simulink model "ModelCtrl"  (R2020b)
settings: Solver=FixedStepAuto  StartTime=0.0  StopTime=15  FixedStep=1/400  RelTol=1e-3
values from neighbouring files (symbols this model uses):
  Df = 0.011 * diag([2 1.9 0.5])    [default_parameters.m]
  fc_m = 5.0    (= 5)    [default_parameters.m]
  g = 9.81    [default_parameters.m]
  INERTIA = diag([1.0 2.0 2.5]) * 1e-4    [default_parameters.m]
  K = [-0.25 0.25 0.25 -0.25 ... (first row only)    [default_parameters.m]
  lb = [0; 0; 0; 0]    [default_parameters.m]
  MASS = 0.85    [default_parameters.m]
  MAX_ANG_ACC = 10 * diag([50.0 50.0 20.0])    [default_parameters.m]
  MAX_ESC_SPD = 6000    [default_parameters.m]
  MAX_TILT_ANGLE = 35.0    (= 35)    [default_parameters.m]
  Thrust_to_grav = 4.0    (= 4)    [default_parameters.m]
  ub = [100.0; 100.0; 100.0; 100.0]    [default_parameters.m]
  W = diag([1.0 1.0 1.0 0.5])    [default_parameters.m]
  wind_spd = [0;0;0]    [default_parameters.m]
undefined symbols (not defined in the file or in its folder): A, B, C, L
libraries: pid_lib x13, sharedtransform x6, aerolibutil x2, shared6dof x1
(part 2 of 2)

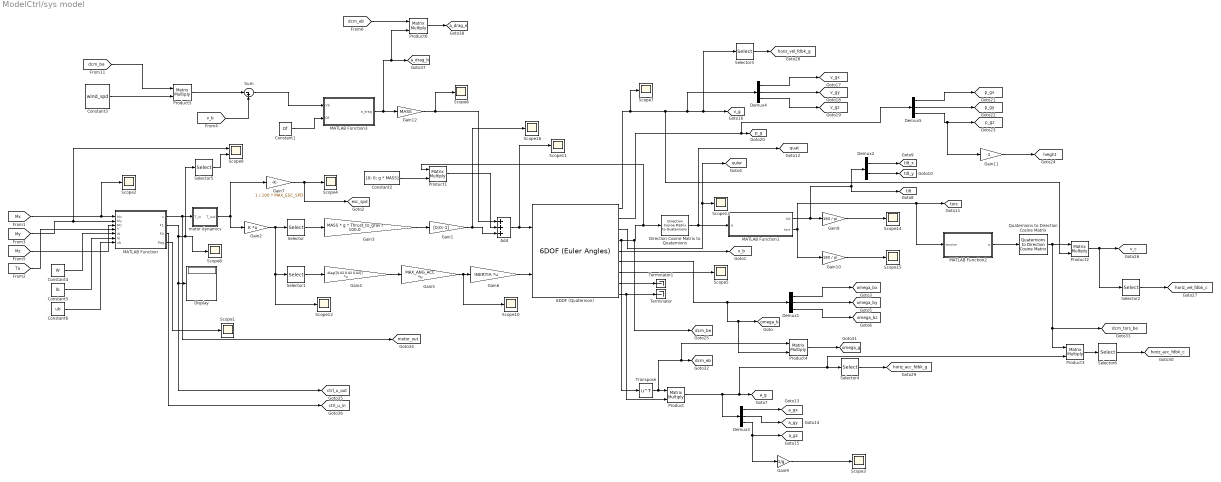
== system ModelCtrl/sys model ==
  6DOF (Quaternion) : shared6dof/6DOF (Euler Angles)  units=Metric (MKS)  mtype=Fixed  rep=Quaternion  xme_0=[0 0 0]  Vm_0=[0 0 0]  eul_0=[0 0 0]  pm_0=[0 0 0]  mass_0=MASS  mass_e=0.5  mass_f=2.0  inertia=INERTIA  inertia_e=eye(3)  inertia_f=2*eye(3)  k_quat=1.0  vre_flag=on  abi_flag=on  aMode=0  xme_statename=''  Vm_statename=''  eul_statename=''  quat_statename=''  pm_statename=''  mass_statename=''
      settings: SourceProductBaseCode=AE,PW,MT,UV,VE,VP
  Add : Sum  Inputs=+++
  Constant1 : Constant  Value=Df
  Constant2 : Constant  Value=[0; 0; g * MASS]
  Constant3 : Constant  Value=wind_spd
  Constant4 : Constant  Value=W
  Constant5 : Constant  Value=lb
  Constant6 : Constant  Value=ub
  Demux{1,3..5} (4 alike) : Demux  Outputs=3
  Demux2 : Demux  Outputs=2
  Direction Cosine Matrix to Quaternions : sharedtransform/Direction Cosine Matrix  to Quaternions  aMode=0  action=None  tolerance=eps(2)
      settings: SourceProductBaseCode=AE,PW,MT,UV,VE,VP
  Display : Display
  Gain1 : Gain  Gain=[0;0;-1]
  Gain10 : Gain  Gain=180 / pi
  Gain11 : Gain  Gain=-1
  Gain12 : Gain  Gain=MASS
  Gain2 : Gain  Gain=K  Multiplication=Matrix(K*u)
  Gain3 : Gain  Gain=MASS * g * Thrust_to_grav / 100.0
  Gain4 : Gain  Gain=diag([0.02 0.02 0.02])  Multiplication=Matrix(K*u)
  Gain5 : Gain  Gain=MAX_ANG_ACC  Multiplication=Matrix(K*u)
  Gain6 : Gain  Gain=INERTIA  Multiplication=Matrix(K*u)
  Gain7 : Gain  Gain=1 / 100 * MAX_ESC_SPD
  Gain8 : Gain  Gain=180 / pi
  Gain9 : Gain  Gain=1/g
  MATLAB Function : MATLAB Function  TreatAsAtomicUnit=on
  MATLAB Function1 : MATLAB Function  TreatAsAtomicUnit=on
  MATLAB Function2 : MATLAB Function  TreatAsAtomicUnit=on
  MATLAB Function3 : MATLAB Function  TreatAsAtomicUnit=on
  Product{,1..6} (7 alike) : Product  Multiplication=Matrix(*)
  Quaternions to Direction Cosine Matrix : sharedtransform/Quaternions to  Direction Cosine Matrix  aMode=aMode
      settings: SourceProductBaseCode=AE,PW,MT,UV,VE,VP
  Scope{1..8,10..16} (15 alike) : Scope
  Scope9 : Scope  NumInputPorts=2
  Selector : Selector  InputPortWidth=4  IndexOptions=Index vector (dialog)  Indices=[4]  OutputSizes=1
  Selector1 : Selector  InputPortWidth=4  IndexOptions=Index vector (dialog)  Indices=[1 2 3]  OutputSizes=1
  Selector{2..4,6} (4 alike) : Selector  InputPortWidth=3  IndexOptions=Index vector (dialog)  Indices=[1 2]  OutputSizes=1
  Selector5 : Selector  InputPortWidth=4  IndexOptions=Index vector (dialog)  Indices=[2]  OutputSizes=1
  Sum : Sum  Inputs=|-+
  Terminator : Terminator
  Terminator1 : Terminator
  Transpose : Math  Operator=transpose  SaturateOnIntegerOverflow=on
  motor dynamics : Subsystem
  tag scope: a_drag_b=global, a_drag_e=global, a_g=global, a_gx=global, a_gy=global, a_gz=global, ctrl_u_in=global, ctrl_u_out=global, dcm_be=global, dcm_eb=global, dcm_tors_be=global, esc_spd=global, euler=global, height=global, horiz_acc_fdbk_c=global, horiz_acc_fdbk_g=global, horiz_vel_fdbk_c=global, horiz_vel_fdbk_g=global, motor_out=global, omega_b=global, omega_bx=global, omega_by=global, omega_bz=global, omega_g=global, p_g=global, p_gx=global, p_gy=global, p_gz=global, quat=global, tilt=global, tilt_x=global, tilt_y=global, tors=global, v_b=global, v_c=global, v_g=global, v_gx=global, v_gy=global, v_gz=global
  wires:
  [Ta] -> MATLAB Function/4(T)
  [My] -> Scope9/1, MATLAB Function/2(My)
  Gain4/1 -> Gain5/1
  Gain2/1 -> Scope12/1, Selector1/1, Selector/1
  Constant5/1 -> MATLAB Function/6(lb)
  Constant6/1 -> MATLAB Function/7(ub)
  motor dynamics/1(T_out) -> Gain7/1, Gain2/1
  6DOF (Quaternion)/5 -> [v_b]
  [Mz] -> MATLAB Function/3(Mz)
  MATLAB Function1/2(tors) -> Gain10/1, MATLAB Function2/1(torsion), [tors]
  Demux1/2 -> [omega_by]
  Selector1/1 -> Gain4/1
  Selector/1 -> Gain3/1
  Demux1/3 -> [omega_bz]
  MATLAB Function/1(x) -> [motor_out], motor dynamics/1(T_in)
  Gain10/1 -> Scope15/1
  6DOF (Quaternion)/4 -> Transpose/1, [dcm_be], Product1/1, Direction Cosine Matrix to Quaternions/1
  Direction Cosine Matrix to Quaternions/1 -> [quat], MATLAB Function1/1(q)
  Gain6/1 -> 6DOF (Quaternion)/2
  [Mx] -> Scope2/1, MATLAB Function/1(Mx)
  Demux1/1 -> [omega_bx]
  6DOF (Quaternion)/3 -> [euler], Scope13/1
  Gain5/1 -> Scope10/1, Gain6/1
  Gain3/1 -> Gain1/1
  MATLAB Function/2(F1) -> [ctrl_u_out], Display/1, Selector5/1, Scope8/1
  MATLAB Function1/1(tilt) -> Demux2/1, [tilt], Gain8/1
  6DOF (Quaternion)/2 -> Demux5/1, [p_g]
  Constant4/1 -> MATLAB Function/5(W)
  Demux2/1 -> [tilt_x]
  Selector5/1 -> Scope9/2
  6DOF (Quaternion)/9 -> Product/2, Terminator/1
  6DOF (Quaternion)/8 -> Terminator1/1
  MATLAB Function/4(flag) -> Scope1/1
  Demux2/2 -> [tilt_y]
  6DOF (Quaternion)/7 -> Scope5/1
  Gain7/1 -> [esc_spd], Scope4/1
  6DOF (Quaternion)/6 -> Product4/2, [omega_b], Demux1/1
  Product/1 -> Demux3/1, Product3/2, Selector4/1, [a_g]
  Demux3/1 -> [a_gx]
  Demux3/2 -> [a_gy]
  Demux3/3 -> Gain9/1, [a_gz]
  Gain9/1 -> Scope3/1
  Gain1/1 -> Scope16/1, Add/3
  Constant2/1 -> Product1/2
  Product1/1 -> Add/2
  Demux4/1 -> [v_gx]
  Demux4/3 -> [v_gz]
  Demux4/2 -> [v_gy]
  Demux5/1 -> [p_gx]
  Demux5/2 -> [p_gy]
  Demux5/3 -> Gain11/1, [p_gz]
  Gain11/1 -> [height]
  MATLAB Function2/1(q) -> Quaternions to Direction Cosine Matrix/1
  Gain8/1 -> Scope14/1
  Quaternions to Direction Cosine Matrix/1 -> [dcm_tors_be], Product3/1, Product2/1
  6DOF (Quaternion)/1 -> Scope7/1, Selector3/1, [v_g], Demux4/1, Product2/2
  Product2/1 -> Selector2/1, [v_c]
  Selector2/1 -> [horiz_vel_fdbk_c]
  Selector3/1 -> [horiz_vel_fdbk_g]
  Selector4/1 -> [horiz_acc_fdbk_g]
  Selector6/1 -> [horiz_acc_fdbk_c]
  Product3/1 -> Selector6/1
  Add/1 -> Scope11/1, 6DOF (Quaternion)/1
  Constant1/1 -> MATLAB Function3/2(Df)
  MATLAB Function3/1(a_drag) -> Product6/2, [a_drag_b], Gain12/1
  Gain12/1 -> Scope6/1, Add/1
  Transpose/1 -> Product4/1, [dcm_eb], Product/1
  Product4/1 -> [omega_g]
  [v_b] -> Sum/2
  [dcm_be] -> Product5/1
  Constant3/1 -> Product5/2
  Product5/1 -> Sum/1
  Sum/1 -> MATLAB Function3/1(Vb)
  MATLAB Function/3(F0) -> [ctrl_u_in]
  [dcm_eb] -> Product6/1
  Product6/1 -> [a_drag_e]

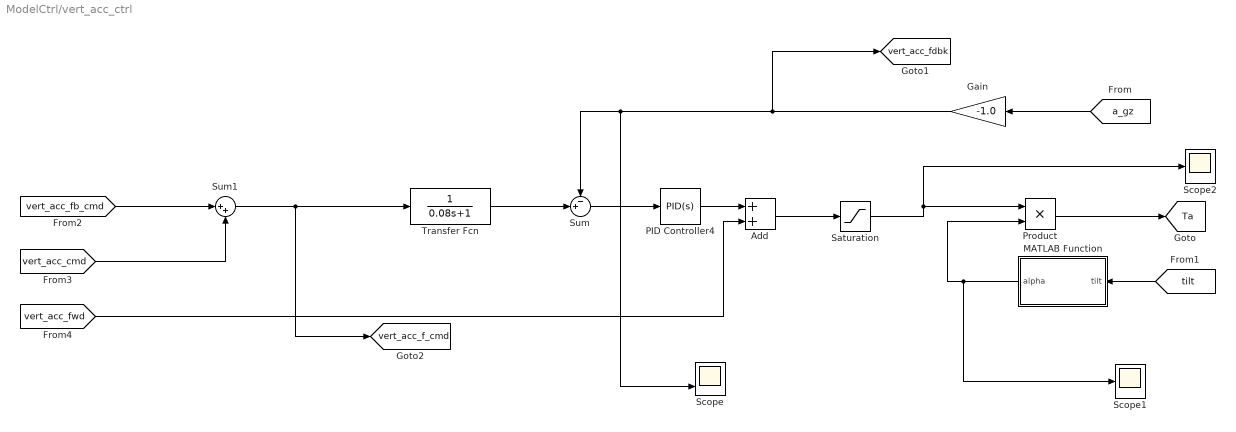
== system ModelCtrl/vert_acc_ctrl ==
  Add : Sum
  Gain : Gain  Gain=-1.0
  MATLAB Function : MATLAB Function  TreatAsAtomicUnit=on
  PID Controller4 : pid_lib/PID Controller  Controller=PID  Form=Ideal  TimeDomain=Continuous-time  UseExternalTs=off  SampleTime=-1  IntegratorMethod=Forward Euler  FilterMethod=Forward Euler  ControllerParametersSource=internal  P=35  I=10  D=0.0  UseFilter=on  N=50  TunerSelectOption=Transfer Function Based (PID Tuner App)  InitialConditionSource=internal  InitialConditionForIntegrator=0  InitialConditionForFilter=0  DifferentiatorICPrevScaledInput=0  ExternalReset=none  TrackingMode=off  Kt=1  LimitOutput=off  SatLimitsSource=internal  UpperSaturationLimit=inf  LowerSaturationLimit=-inf  LinearizeAsGain=on  AntiWindupMode=none  Kb=1  POutMin=[]  POutMax=[]  IOutMin=[]  IOutMax=[]  DOutMin=[]  DOutMax=[]  NOutMin=[]  NOutMax=[]  SumOutMin=[]  SumOutMax=[]  SaturationOutMin=[]  SaturationOutMax=[]  PParamMin=[]  PParamMax=[]  IParamMin=[]  IParamMax=[]  DParamMin=[]  DParamMax=[]  NParamMin=[]  NParamMax=[]  KbParamMin=[]  KbParamMax=[]  KtParamMin=[]  KtParamMax=[]  KbOutMin=[]  KbOutMax=[]  KtOutMin=[]  KtOutMax=[]  IntegratorOutMin=[]  IntegratorOutMax=[]  FilterOutMin=[]  FilterOutMax=[]  SumI1OutMin=[]  SumI1OutMax=[]  SumI2OutMin=[]  SumI2OutMax=[]  SumI3OutMin=[]  SumI3OutMax=[]  SumI4OutMin=[]  SumI4OutMax=[]  SumDOutMin=[]  SumDOutMax=[]  DifferentiatorOutMin=[]  DifferentiatorOutMax=[]  FilterDiffOutCoefMin=[]  FilterDiffOutCoefMax=[]  ReciprocalOutMin=[]  ReciprocalOutMax=[]  SumDenOutMin=[]  SumDenOutMax=[]  SumNumOutMin=[]  SumNumOutMax=[]  DivideOutMin=[]  DivideOutMax=[]  UdiffTsProdOutMin=[]  UdiffTsProdOutMax=[]  NTsProdOutMin=[]  NTsProdOutMax=[]  UintegralTsProdOutMin=[]  UintegralTsProdOutMax=[]  UngainTsProdOutMin=[]  UngainTsProdOutMax=[]  IntegratorContinuousStateAttributes=''  IntegratorStateMustResolveToSignalObject=off  IntegratorRTWStateStorageClass=Auto  FilterContinuousStateAttributes=''  FilterStateMustResolveToSignalObject=off  FilterRTWStateStorageClass=Auto  ParallelPVariant=Passthrough  IdealPVariant=InternalParameters  IVariant=InternalParameters  DVariant=InternalParameters  IntegratorVariant=Continuous  SatVariant=Disabled  AWVariant=Passthrough  PCopyVariant=Disabled  TRVariant=Disabled  FdbkBlocksVariant=Forward  IdealPFdbkVariant=Disabled  SatFdbkVariant=Disabled  DerivativeFilterVariant=ContFilter  NVariant=InternalParameters  NCopyVariant=Disabled  FilterICVariant=InternalICsFilter  IntegratorICVariant=InternalICs  ExternalResetVariant=Disabled  TRSumVariant=Passthrough  SumFdbkVariant=Disabled  SumVariant=Sum_PID  TsampFilterVariant=InternalTs  TsampNgainVariant=Passthrough  TsampIntegralVariant=Passthrough  ExternalSaturationOutDataTypeStr=Inherit: Same as second input
  Product : Product
  Saturation : Saturate  UpperLimit=100  LowerLimit=0
  Scope : Scope  NumInputPorts=2
  Scope1 : Scope
  Scope2 : Scope
  Sum : Sum  Inputs=-+|
  Sum1 : Sum  Inputs=|++
  Transfer Fcn : TransferFcn  Denominator=[0.08 1]
  tag scope: Ta=global, vert_acc_f_cmd=global, vert_acc_fdbk=global
  wires:
  [a_gz] -> Gain/1
  Sum/1 -> PID Controller4/1
  Gain/1 -> [vert_acc_fdbk], Sum/1, Scope/2
  [tilt] -> MATLAB Function/1(tilt)
  MATLAB Function/1(alpha) -> Scope1/1, Product/2
  Product/1 -> [Ta]
  Transfer Fcn/1 -> Sum/2
  Saturation/1 -> Scope2/1, Product/1
  PID Controller4/1 -> Add/1
  Add/1 -> Saturation/1
  [vert_acc_fb_cmd] -> Sum1/1
  [vert_acc_cmd] -> Sum1/2
  Sum1/1 -> [vert_acc_f_cmd], Transfer Fcn/1
  [vert_acc_fwd] -> Add/2

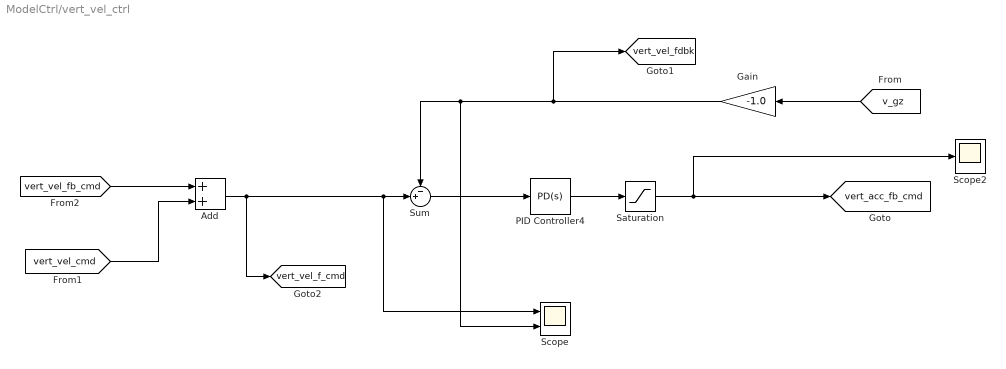
== system ModelCtrl/vert_vel_ctrl ==
  Add : Sum
  Gain : Gain  Gain=-1.0
  PID Controller4 : pid_lib/PID Controller  Controller=PD  Form=Ideal  TimeDomain=Continuous-time  UseExternalTs=off  SampleTime=-1  IntegratorMethod=Forward Euler  FilterMethod=Forward Euler  ControllerParametersSource=internal  P=5  I=1.5  D=0.02  UseFilter=on  N=50  TunerSelectOption=Transfer Function Based (PID Tuner App)  InitialConditionSource=internal  InitialConditionForIntegrator=0  InitialConditionForFilter=0  DifferentiatorICPrevScaledInput=0  ExternalReset=none  TrackingMode=off  Kt=1  LimitOutput=off  SatLimitsSource=internal  UpperSaturationLimit=inf  LowerSaturationLimit=-inf  LinearizeAsGain=on  AntiWindupMode=none  Kb=1  POutMin=[]  POutMax=[]  IOutMin=[]  IOutMax=[]  DOutMin=[]  DOutMax=[]  NOutMin=[]  NOutMax=[]  SumOutMin=[]  SumOutMax=[]  SaturationOutMin=[]  SaturationOutMax=[]  PParamMin=[]  PParamMax=[]  IParamMin=[]  IParamMax=[]  DParamMin=[]  DParamMax=[]  NParamMin=[]  NParamMax=[]  KbParamMin=[]  KbParamMax=[]  KtParamMin=[]  KtParamMax=[]  KbOutMin=[]  KbOutMax=[]  KtOutMin=[]  KtOutMax=[]  IntegratorOutMin=[]  IntegratorOutMax=[]  FilterOutMin=[]  FilterOutMax=[]  SumI1OutMin=[]  SumI1OutMax=[]  SumI2OutMin=[]  SumI2OutMax=[]  SumI3OutMin=[]  SumI3OutMax=[]  SumI4OutMin=[]  SumI4OutMax=[]  SumDOutMin=[]  SumDOutMax=[]  DifferentiatorOutMin=[]  DifferentiatorOutMax=[]  FilterDiffOutCoefMin=[]  FilterDiffOutCoefMax=[]  ReciprocalOutMin=[]  ReciprocalOutMax=[]  SumDenOutMin=[]  SumDenOutMax=[]  SumNumOutMin=[]  SumNumOutMax=[]  DivideOutMin=[]  DivideOutMax=[]  UdiffTsProdOutMin=[]  UdiffTsProdOutMax=[]  NTsProdOutMin=[]  NTsProdOutMax=[]  UintegralTsProdOutMin=[]  UintegralTsProdOutMax=[]  UngainTsProdOutMin=[]  UngainTsProdOutMax=[]  IntegratorContinuousStateAttributes=''  IntegratorStateMustResolveToSignalObject=off  IntegratorRTWStateStorageClass=Auto  FilterContinuousStateAttributes=''  FilterStateMustResolveToSignalObject=off  FilterRTWStateStorageClass=Auto  ParallelPVariant=Passthrough  IdealPVariant=InternalParameters  IVariant=Disabled  DVariant=InternalParameters  IntegratorVariant=Disabled  SatVariant=Disabled  AWVariant=Disabled  PCopyVariant=Disabled  TRVariant=Disabled  FdbkBlocksVariant=Forward  IdealPFdbkVariant=Disabled  SatFdbkVariant=Disabled  DerivativeFilterVariant=ContFilter  NVariant=InternalParameters  NCopyVariant=Disabled  FilterICVariant=InternalICsFilter  IntegratorICVariant=Disabled  ExternalResetVariant=Disabled  TRSumVariant=Passthrough  SumFdbkVariant=Disabled  SumVariant=Sum_PD  TsampFilterVariant=InternalTs  TsampNgainVariant=Passthrough  TsampIntegralVariant=Disabled_SignalSpec  ExternalSaturationOutDataTypeStr=Inherit: Same as second input
  Saturation : Saturate  UpperLimit=8  LowerLimit=-8
  Scope : Scope  NumInputPorts=2
  Scope2 : Scope
  Sum : Sum  Inputs=-+|
  tag scope: vert_acc_fb_cmd=global, vert_vel_f_cmd=global, vert_vel_fdbk=global
  wires:
  [v_gz] -> Gain/1
  Sum/1 -> PID Controller4/1
  Gain/1 -> [vert_vel_fdbk], Sum/1, Scope/2
  PID Controller4/1 -> Saturation/1
  Saturation/1 -> [vert_acc_fb_cmd], Scope2/1
  Add/1 -> [vert_vel_f_cmd], Scope/1, Sum/2
  [vert_vel_fb_cmd] -> Add/1
  [vert_vel_cmd] -> Add/2

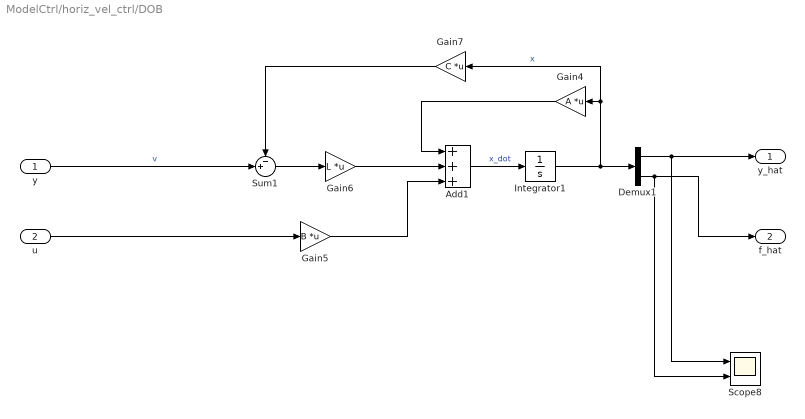
== system ModelCtrl/horiz_vel_ctrl/DOB ==
  y : Inport
  u : Inport  Port=2
  Add1 : Sum  Inputs=+++
  Demux1 : Demux  Outputs=2
  Gain4 : Gain  Gain=A  Multiplication=Matrix(K*u)
  Gain5 : Gain  Gain=B  Multiplication=Matrix(K*u)
  Gain6 : Gain  Gain=L  Multiplication=Matrix(K*u)
  Gain7 : Gain  Gain=C  Multiplication=Matrix(K*u)
  Integrator1 : Integrator
  Scope8 : Scope  NumInputPorts=2
  Sum1 : Sum  Inputs=-+|
  y_hat : Outport
  f_hat : Outport  Port=2
  wires:
  Gain4/1 -> Add1/1
  Integrator1/1 -> Demux1/1, Gain7/1, Gain4/1  "x"
  y/1 -> Sum1/2  "v"
  Add1/1 -> Integrator1/1  "x_dot"
  Gain7/1 -> Sum1/1
  Gain6/1 -> Add1/2
  Sum1/1 -> Gain6/1
  Gain5/1 -> Add1/3
  u/1 -> Gain5/1
  Demux1/1 -> Scope8/1, y_hat/1
  Demux1/2 -> Scope8/2, f_hat/1

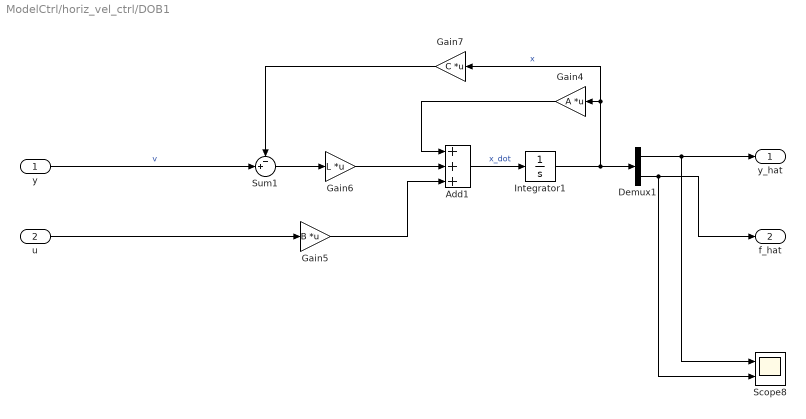
== system ModelCtrl/horiz_vel_ctrl/DOB1 ==
  y : Inport
  u : Inport  Port=2
  Add1 : Sum  Inputs=+++
  Demux1 : Demux  Outputs=2
  Gain4 : Gain  Gain=A  Multiplication=Matrix(K*u)
  Gain5 : Gain  Gain=B  Multiplication=Matrix(K*u)
  Gain6 : Gain  Gain=L  Multiplication=Matrix(K*u)
  Gain7 : Gain  Gain=C  Multiplication=Matrix(K*u)
  Integrator1 : Integrator
  Scope8 : Scope  NumInputPorts=2
  Sum1 : Sum  Inputs=-+|
  y_hat : Outport
  f_hat : Outport  Port=2
  wires:
  Gain4/1 -> Add1/1
  Integrator1/1 -> Demux1/1, Gain7/1, Gain4/1  "x"
  y/1 -> Sum1/2  "v"
  Add1/1 -> Integrator1/1  "x_dot"
  Gain7/1 -> Sum1/1
  Gain6/1 -> Add1/2
  Sum1/1 -> Gain6/1
  Gain5/1 -> Add1/3
  u/1 -> Gain5/1
  Demux1/1 -> Scope8/1, y_hat/1
  Demux1/2 -> Scope8/2, f_hat/1

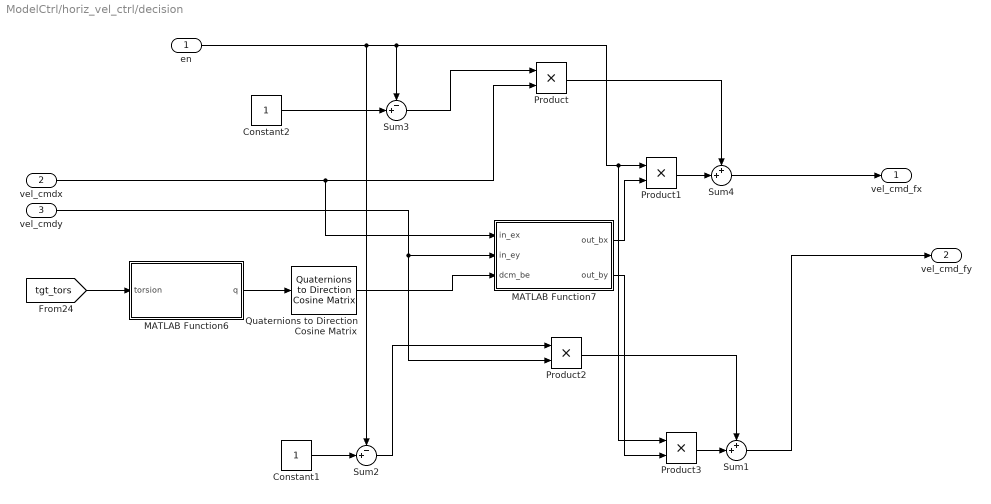
== system ModelCtrl/horiz_vel_ctrl/decision ==
  en : Inport
  vel_cmdx : Inport  Port=2
  vel_cmdy : Inport  Port=3
  Constant1 : Constant
  Constant2 : Constant
  MATLAB Function6 : MATLAB Function  TreatAsAtomicUnit=on
  MATLAB Function7 : MATLAB Function  TreatAsAtomicUnit=on
  Product{,1..3} (4 alike) : Product
  Quaternions to Direction Cosine Matrix : sharedtransform/Quaternions to  Direction Cosine Matrix  aMode=aMode
      settings: SourceProductBaseCode=AE,PW,MT,UV,VE,VP
  Sum1 : Sum  Inputs=++|
  Sum2 : Sum  Inputs=-+|
  Sum3 : Sum  Inputs=-+|
  Sum4 : Sum  Inputs=++|
  vel_cmd_fx : Outport
  vel_cmd_fy : Outport  Port=2
  wires:
  vel_cmdx/1 -> MATLAB Function7/1(in_ex), Product/2
  Product/1 -> Sum4/1
  Product1/1 -> Sum4/2
  Sum4/1 -> vel_cmd_fx/1
  MATLAB Function6/1(q) -> Quaternions to Direction Cosine Matrix/1
  [tgt_tors] -> MATLAB Function6/1(torsion)
  Quaternions to Direction Cosine Matrix/1 -> MATLAB Function7/3(dcm_be)
  vel_cmdy/1 -> Product2/2, MATLAB Function7/2(in_ey)
  MATLAB Function7/1(out_bx) -> Product1/2
  Constant1/1 -> Sum2/2
  Product3/1 -> Sum1/2
  Product2/1 -> Sum1/1
  MATLAB Function7/2(out_by) -> Product3/2
  Sum1/1 -> vel_cmd_fy/1
  en/1 -> Sum2/1, Sum3/1, Product3/1, Product1/1
  Constant2/1 -> Sum3/2
  Sum3/1 -> Product/1
  Sum2/1 -> Product2/1

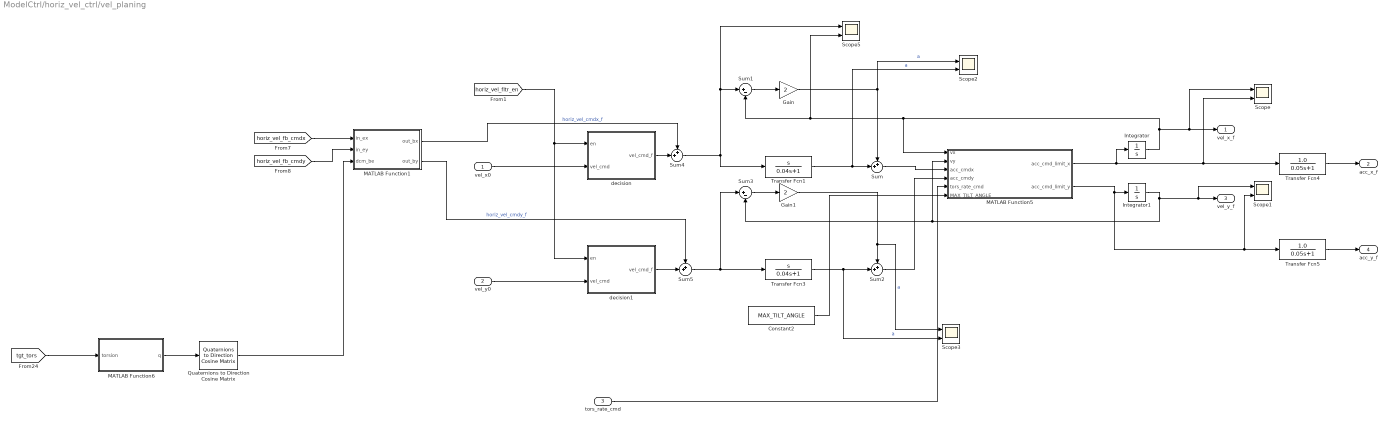
== system ModelCtrl/horiz_vel_ctrl/vel_planing ==
  vel_x0 : Inport
  vel_y0 : Inport  Port=2
  tors_rate_cmd : Inport  Port=3
  Constant2 : Constant  Value=MAX_TILT_ANGLE
  Gain : Gain  Gain=2
  Gain1 : Gain  Gain=2
  Integrator : Integrator
  Integrator1 : Integrator
  MATLAB Function1 : MATLAB Function  TreatAsAtomicUnit=on
  MATLAB Function5 : MATLAB Function  TreatAsAtomicUnit=on
  MATLAB Function6 : MATLAB Function  TreatAsAtomicUnit=on
  Quaternions to Direction Cosine Matrix : sharedtransform/Quaternions to  Direction Cosine Matrix  aMode=aMode
      settings: SourceProductBaseCode=AE,PW,MT,UV,VE,VP
  Scope{,1..3,5} (5 alike) : Scope  NumInputPorts=2
  Sum{,2,4..5} (4 alike) : Sum  Inputs=++|
  Sum1 : Sum  Inputs=|+-
  Sum3 : Sum  Inputs=|+-
  Transfer Fcn1 : TransferFcn  Numerator=[1 0]  Denominator=[0.04 1]
  Transfer Fcn3 : TransferFcn  Numerator=[1 0]  Denominator=[0.04 1]
  Transfer Fcn4 : TransferFcn  Numerator=[1.0]  Denominator=[0.05 1]
  Transfer Fcn5 : TransferFcn  Numerator=[1.0]  Denominator=[0.05 1]
  decision : Subsystem
  decision1 : Subsystem
  vel_x_f : Outport
  acc_x_f : Outport  Port=2
  vel_y_f : Outport  Port=3
  acc_y_f : Outport  Port=4
  wires:
  Transfer Fcn3/1 -> Scope3/2, Sum2/2  "a"
  Integrator/1 -> Scope5/2, Sum1/2, MATLAB Function5/1(vx), Scope/1, vel_x_f/1
  Integrator1/1 -> Scope1/1, vel_y_f/1, Sum3/2, MATLAB Function5/2(vy)
  Sum/1 -> MATLAB Function5/3(acc_cmdx)
  Sum5/1 -> Sum3/1, Transfer Fcn3/1
  Sum1/1 -> Gain/1
  Sum3/1 -> Gain1/1
  Sum2/1 -> MATLAB Function5/4(acc_cmdy)
  Transfer Fcn1/1 -> Scope2/2, Sum/2  "a"
  vel_y0/1 -> decision1/2(vel_cmd)
  Constant2/1 -> MATLAB Function5/6(MAX_TILT_ANGLE)
  MATLAB Function5/1(acc_cmd_limit_x) -> Integrator/1, Scope/2, Transfer Fcn4/1
  MATLAB Function5/2(acc_cmd_limit_y) -> Scope1/2, Transfer Fcn5/1, Integrator1/1
  Transfer Fcn5/1 -> acc_y_f/1
  Transfer Fcn4/1 -> acc_x_f/1
  Gain/1 -> Sum/1, Scope2/1  "a"
  Gain1/1 -> Scope3/1, Sum2/1  "a"
  tors_rate_cmd/1 -> MATLAB Function5/5(tors_rate_cmd)
  Sum4/1 -> Scope5/1, Sum1/1, Transfer Fcn1/1
  [horiz_vel_fltr_en] -> decision1/1(en), decision/1(en)
  vel_x0/1 -> decision/2(vel_cmd)
  decision/1(vel_cmd_f) -> Sum4/2
  [horiz_vel_fb_cmdx] -> MATLAB Function1/1(in_ex)
  [horiz_vel_fb_cmdy] -> MATLAB Function1/2(in_ey)
  MATLAB Function6/1(q) -> Quaternions to Direction Cosine Matrix/1
  [tgt_tors] -> MATLAB Function6/1(torsion)
  Quaternions to Direction Cosine Matrix/1 -> MATLAB Function1/3(dcm_be)
  MATLAB Function1/1(out_bx) -> Sum4/1  "horiz_vel_cmdx_f"
  decision1/1(vel_cmd_f) -> Sum5/2
  MATLAB Function1/2(out_by) -> Sum5/1  "horiz_vel_cmdy_f"

== system ModelCtrl/sys model/motor dynamics ==
  T_in : Inport
  Demux : Demux
  Mux : Mux
  Transfer Fcn{,1..3} (4 alike) : TransferFcn  Denominator=[1/(2*pi*fc_m) 1]
  T_out : Outport
  wires:
  Transfer Fcn3/1 -> Mux/4
  Transfer Fcn2/1 -> Mux/3
  Demux/2 -> Transfer Fcn1/1
  Demux/4 -> Transfer Fcn3/1
  Demux/1 -> Transfer Fcn/1
  Transfer Fcn1/1 -> Mux/2
  Transfer Fcn/1 -> Mux/1
  Demux/3 -> Transfer Fcn2/1
  Mux/1 -> T_out/1  "T_out"
  T_in/1 -> Demux/1

== system ModelCtrl/horiz_vel_ctrl/vel_planing/decision ==
  en : Inport
  vel_cmd : Inport  Port=2
  Constant : Constant
  Product : Product
  Product1 : Product
  Sum4 : Sum  Inputs=++|
  Sum5 : Sum  Inputs=-+|
  Transfer Fcn : TransferFcn  Denominator=[1.2 1]
  vel_cmd_f : Outport
  wires:
  Transfer Fcn/1 -> Product1/2
  en/1 -> Product1/1, Sum5/1
  vel_cmd/1 -> Product/2, Transfer Fcn/1
  Sum5/1 -> Product/1
  Product/1 -> Sum4/1
  Product1/1 -> Sum4/2
  Constant/1 -> Sum5/2
  Sum4/1 -> vel_cmd_f/1

== system ModelCtrl/horiz_vel_ctrl/vel_planing/decision1 ==
  en : Inport
  vel_cmd : Inport  Port=2
  Constant : Constant
  Product : Product
  Product1 : Product
  Sum4 : Sum  Inputs=++|
  Sum5 : Sum  Inputs=-+|
  Transfer Fcn : TransferFcn  Denominator=[1.2 1]
  vel_cmd_f : Outport
  wires:
  Transfer Fcn/1 -> Product1/2
  en/1 -> Product1/1, Sum5/1
  vel_cmd/1 -> Product/2, Transfer Fcn/1
  Sum5/1 -> Product/1
  Product/1 -> Sum4/1
  Product1/1 -> Sum4/2
  Constant/1 -> Sum5/2
  Sum4/1 -> vel_cmd_f/1

== matlab function ModelCtrl/horiz_vel_ctrl/MATLAB Function6 ==
  data: torsion input; q output
function q = tors_to_quat(torsion)
q = zeros(4,1);
q(1) = cos(torsion / 2.0);
q(2) = 0.0;
q(3) = 0.0;
q(4) = sin(torsion / 2.0);

== matlab function ModelCtrl/horiz_vel_ctrl/MATLAB Function7 ==
  data: out_bx output; in_ex input; in_ey input; dcm_be input; out_by output
function [out_bx, out_by] = e_to_b_2d(in_ex, in_ey, dcm_be)
y = dcm_be * [in_ex; in_ey; 0];
out_bx = y(1);
out_by = y(2);

== matlab function ModelCtrl/horiz_vel_ctrl/MATLAB Function3 ==
  data: Vbx input; Vby input; a_drag_x output; Df input; a_drag_y output
function [a_drag_x, a_drag_y]  = drag_from_vb(Vbx, Vby, Df)
Vb = [Vbx; Vby; 0];
W = diag(sign(Vb));
a_drag = W * Df * Vb.^2;
a_drag_x = a_drag(1);
a_drag_y = a_drag(2);

== matlab function ModelCtrl/horiz_vel_ctrl/MATLAB Function5 ==
  data: max_tilt input; tilt_cmd_limit output; tilt_cmd input
function tilt_cmd_limit = limit_tilt_cmd(max_tilt, tilt_cmd)
tilt_norm = norm(tilt_cmd);
if tilt_norm > max_tilt
    tilt_cmd_limit = tilt_cmd / tilt_norm * max_tilt;
else
    tilt_cmd_limit = tilt_cmd;
end

== matlab function ModelCtrl/ang_vel_ctrl/MATLAB Function4 ==
  data: max_ang_vel_cmd input; ang_limit_cmdx output; wx input; wy input; wz input; ang_limit_cmdy output; ang_limit_cmdz output
function [ang_limit_cmdx, ang_limit_cmdy, ang_limit_cmdz] = limit_ang_vel_cmd(max_ang_vel_cmd, wx, wy, wz)
if norm([wx wy]) > max_ang_vel_cmd(1)
    horiz_cmd_limit = [wx wy] / norm([wx wy]) * max_ang_vel_cmd(1);
else
    horiz_cmd_limit = [wx wy];
end
ang_limit_cmdx = horiz_cmd_limit(1);
ang_limit_cmdy = horiz_cmd_limit(2);

if norm(wz) > max_ang_vel_cmd(2)
    ang_limit_cmdz = wz / norm(wz) * max_ang_vel_cmd(2);
else
    ang_limit_cmdz = wz;
end

== matlab function ModelCtrl/horiz_vel_ctrl/vel_planing/MATLAB Function5 ==
  data: acc_cmd_limit_x output; vx input; vy input; acc_cmdx input; acc_cmdy input; tors_rate_cmd input; acc_cmd_limit_y output; MAX_TILT_ANGLE input
function [acc_cmd_limit_x, acc_cmd_limit_y] = limit_acc_cmd(vx, vy, acc_cmdx, acc_cmdy, tors_rate_cmd, MAX_TILT_ANGLE)
v_a = [vx; vy];
acc_cmd = [acc_cmdx; acc_cmdy];
r = tand(MAX_TILT_ANGLE) * 9.81;
vel_t = [0.0000    5.4947    8.5657   10.9229   13.0248   15.0724   17.1915   19.4878];
atti_t = [0     5    10    15    20    25    30    35];
acc_t = 9.81 * tand(atti_t);

v_norm = norm(v_a);

if v_norm > eps
    a_norm = interp1(vel_t, acc_t, v_norm);
    tmp = cross([0;0;tors_rate_cmd], [v_a;0]);
    acc = a_norm * v_a / v_norm + tmp(1:2);
    a = acc(1);
    b = acc(2);
else
    a = 0.0;
    b = 0.0;
end

x0 = acc_cmd(1);
y0 = acc_cmd(2);
x = x0;
y = y0;
x1 = 0;
x2 = 0;
y1 = 0;
y2 = 0;

if (x0 + a)^2 + (y0 + b)^2 > r^2
    % case 1: y = k1 * x (k1 is not inf)    
    if abs(x0) > eps
        k1 = y0 / x0;
        A = k1^2 + 1;
        B = 2 * a + 2 * k1 * b;
        C = a^2 + b^2 - r^2;
        x1 = (-B + sqrt(B^2 - 4 * A * C))/ (2 * A);
        x2 = (-B - sqrt(B^2 - 4 * A * C))/ (2 * A);
        y1 = k1 * x1;
        y2 = k1 * x2;
    % case 2: x = k2 * y (k2 is not inf)   
    elseif abs(y0) > eps
        k2 = x0 / y0;
        A = k2^2 + 1;
        B = 2 * b + 2 * k2 * a;
        C = a^2 + b^2 - r^2;
        y1 = (-B + sqrt(B^2 - 4 * A * C))/ (2 * A);
        y1 = (-B - sqrt(B^2 - 4 * A * C))/ (2 * A);
        x1 = k2 * y1;
        x2 = k2 * y2;
    end
    d1 = norm([x1 y1] - [x0 y0]);
    d2 = norm([x2 y2] - [x0 y0]);
    
    if d1 < d2
        x = x1;
        y = y1;
    else
        x = x2;
        y = y2;
    end
    acc_cmd_limit = [x;y];
else
    acc_cmd_limit = acc_cmd;
end

acc_cmd_limit_x = acc_cmd_limit(1);
acc_cmd_limit_y = acc_cmd_limit(2);

== matlab function ModelCtrl/sys model/MATLAB Function1 ==
  data: q input; tilt output; tors output
function [tilt, tors] = tors_tilt_from_quat(q)
q = q .* [1; -1; -1; -1];

tmp = sqrt(q(1)^2 + q(4)^2);
if tmp < 1e-4
    q_tilt = [0; 1; 0; 0];
    q_tors = [1; 0; 0; 0];
else
    q_tilt = [tmp; 
            (q(1) * q(2) - q(3) * q(4)) / tmp;
            (q(1) * q(3) + q(2) * q(4)) / tmp;
            0];
    q_tors = [q(1) / tmp; 0; 0; q(4) / tmp];
end

q_tilt = q_tilt / norm(q_tilt);
q_tors = q_tors / norm(q_tors);

q_tilt = q_tilt .* [1; -1; -1; -1]; 
q_tors = q_tors .* [1; -1; -1; -1]; 


cos_half_theta = q_tilt(1);
if abs(cos_half_theta - 1.0) < eps
    tilt = [0; 0];
else
    sin_half_theta = sqrt(q_tilt(2)^2 + q_tilt(3)^2);
    theta = 2.0 * atan2(sin_half_theta, cos_half_theta);
    tilt_axis = [q_tilt(2);q_tilt(3)];
    tilt_axis = tilt_axis / norm(tilt_axis);
    tilt = theta * tilt_axis;
end
tors = 2.0 * atan2(q_tors(4), q_tors(1));

== matlab function ModelCtrl/horiz_vel_ctrl/MATLAB Function1 ==
  data: out_bx output; in_ex input; in_ey input; dcm_be input; out_by output
function [out_bx, out_by] = e_to_b_2d(in_ex, in_ey, dcm_be)
y = dcm_be * [in_ex; in_ey; 0];
out_bx = y(1);
out_by = y(2);

== matlab function ModelCtrl/horiz_vel_ctrl/MATLAB Function8 ==
  data: Vbx input; Vby input; a_cent_x output; tors_rate_cmd input; a_cent_y output
function [a_cent_x, a_cent_y]  = cent_d_from_vb(Vbx, Vby, tors_rate_cmd)
tmp = cross([0;0;tors_rate_cmd], [Vbx;Vby;0]);
a_cent_x = tmp(1);
a_cent_y = tmp(2);

== matlab function ModelCtrl/atti_ctrl/MATLAB Function1 ==
  data: tors_ctrl_en input; tors_ctrl_enable output; tors_rate_cmd input
function tors_ctrl_enable = tors_ctrl(tors_ctrl_en, tors_rate_cmd)
tors_ctrl_enable = tors_ctrl_en;
if abs(tors_rate_cmd) < eps
    tors_ctrl_enable = 1.0;
end

== matlab function ModelCtrl/horiz_vel_ctrl/vel_planing/MATLAB Function1 ==
  data: out_bx output; in_ex input; in_ey input; dcm_be input; out_by output
function [out_bx, out_by] = e_to_b_2d(in_ex, in_ey, dcm_be)
y = dcm_be * [in_ex; in_ey; 0];
out_bx = y(1);
out_by = y(2);

== matlab function ModelCtrl/horiz_vel_ctrl/decision/MATLAB Function6 ==
  data: torsion input; q output
function q = tors_to_quat(torsion)
q = zeros(4,1);
q(1) = cos(torsion / 2.0);
q(2) = 0.0;
q(3) = 0.0;
q(4) = sin(torsion / 2.0);

== matlab function ModelCtrl/horiz_vel_ctrl/decision/MATLAB Function7 ==
  data: out_bx output; in_ex input; in_ey input; dcm_be input; out_by output
function [out_bx, out_by] = b_to_e_2d(in_ex, in_ey, dcm_be)
y = dcm_be' * [in_ex; in_ey; 0];
out_bx = y(1);
out_by = y(2);

== matlab function ModelCtrl/horiz_vel_ctrl/vel_planing/MATLAB Function6 ==
  data: torsion input; q output
function q = tors_to_quat(torsion)
q = zeros(4,1);
q(1) = cos(torsion / 2.0);
q(2) = 0.0;
q(3) = 0.0;
q(4) = sin(torsion / 2.0);

== matlab function ModelCtrl/sys model/MATLAB Function ==
  data: Mx input; My input; Mz input; T input; x output; W input; lb input; ub input; F1 output; F0 output; flag output
function [x, F1, F0, flag] = mixer_solver(Mx, My, Mz, T, W, lb, ub)
K = [-0.25 0.25 0.25 -0.25;
     0.25 0.25 -0.25 -0.25;
     0.25 -0.25 0.25 -0.25;
     0.25 0.25 0.25 0.25];
F = [Mx; My; Mz; T];
F0 = F;
P = 2 * K' * W * K;
q = (-2 * K' * W * F);

opts = optimoptions('quadprog','Algorithm','active-set');
x0 = [0;0;0;0];
x = quadprog(P,q,[],[],[],[],lb,ub,x0,opts);
F1 = K * x;

if norm(F - F1) > 0.001
    flag = 1;
else
    flag = 0;
end

== matlab function ModelCtrl/atti_ctrl/MATLAB Function2 ==
  data: tiltx input; q_tilt output; tilty input
function q_tilt = tilt_to_quat(tiltx, tilty)
tilt = [tiltx; tilty];
q_tilt = zeros(4,1);
theta = norm(tilt);
if abs(theta) < eps
    n = [0; 0];
else
    n = tilt / theta;
end
q_tilt(1) = cos(theta / 2.0);
q_tilt(2) = n(1) * sin(theta / 2.0);
q_tilt(3) = n(2) * sin(theta / 2.0);
q_tilt(4) = 0;

== matlab function ModelCtrl/atti_ctrl/MATLAB Function3 ==
  data: torsion input; q_tors output
function q_tors = tors_to_quat(torsion)
q_tors = zeros(4,1);
q_tors(1) = cos(torsion / 2.0);
q_tors(2) = 0.0;
q_tors(3) = 0.0;
q_tors(4) = sin(torsion / 2.0);

== matlab function ModelCtrl/atti_ctrl/MATLAB Function4 ==
  data: q input; tilt output; tors output
function [tilt, tors] = tilt_tors_from_quat(q)
q = [q(1); q(2); q(3); q(4)];

tmp = sqrt(q(1)^2 + q(4)^2);
if tmp < eps
    q_tilt = [0; 1; 0; 0];
    q_tors = [1; 0; 0; 0];
else
    q_tilt = [tmp; 
            (q(1) * q(2) - q(3) * q(4)) / tmp;
            (q(1) * q(3) + q(2) * q(4)) / tmp;
            0];
    q_tors = [q(1) / tmp; 0; 0; q(4) / tmp];
end

q_tilt = q_tilt / norm(q_tilt);
q_tors = q_tors / norm(q_tors);

cos_half_theta = q_tilt(1);
if abs(cos_half_theta - 1.0) < eps
    tilt = [0; 0];
else
    sin_half_theta = sqrt(q_tilt(2)^2 + q_tilt(3)^2);
    theta = 2.0 * atan2(sin_half_theta, cos_half_theta);
    tilt_axis = [q_tilt(2);q_tilt(3)];
    tilt_axis = tilt_axis / norm(tilt_axis);
    tilt = theta * tilt_axis;
end
tors = 2.0 * atan2(q_tors(4), q_tors(1));

== matlab function ModelCtrl/vert_acc_ctrl/MATLAB Function ==
  data: tilt input; alpha output
function alpha = tilt_cmp(tilt)
alpha = 1.0 / cos(norm(tilt));

== matlab function ModelCtrl/sys model/MATLAB Function2 ==
  data: torsion input; q output
function q = tors_to_quat(torsion)
q = zeros(4,1);
q(1) = cos(torsion / 2.0);
q(2) = 0.0;
q(3) = 0.0;
q(4) = sin(torsion / 2.0);

== matlab function ModelCtrl/sys model/MATLAB Function3 ==
  data: Vb input; a_drag output; Df input
function a_drag  = drag_from_vb(Vb, Df)
W = -diag(sign(Vb));
a_drag = W * Df * Vb.^2;

== matlab function ModelCtrl/horiz_vel_ctrl/MATLAB Function4 ==
  data: horiz_acc_x input; horiz_acc_y input; dcm_be output; vert_acc input
function dcm_be = dcm_be_from_acc_cmd(horiz_acc_x, horiz_acc_y, vert_acc)
g = 9.81;
horiz_acc = [horiz_acc_x; horiz_acc_y];
a_tilt = [horiz_acc;-vert_acc] - [0;0;g];
x = [0;0;-1];
norm_a_tilt = norm(a_tilt);

if norm_a_tilt < eps
    x1 = x;
else
    x1 = a_tilt / norm_a_tilt;
end

tmp = cross(x, x1);
if abs(tmp) < eps
    dcm = eye(3);
else 
    sin_theta = norm(tmp);
    axis = tmp / sin_theta;
    cos_theta = dot(x, x1);
%     theta = atan2(sin_theta, cos_theta);
    axis_skew = [0 -axis(3) axis(2);
                 axis(3) 0 -axis(1);
                 -axis(2) axis(1) 0];
    dcm = eye(3) + axis_skew * sin_theta + axis_skew^2 * (1 - cos_theta);
end
dcm_be = dcm';

== matlab function ModelCtrl/horiz_vel_ctrl/MATLAB Function2 ==
  data: q input; tilt output; tors output
function [tilt, tors] = tors_tilt_from_quat(q)
q = q .* [1; -1; -1; -1];

tmp = sqrt(q(1)^2 + q(4)^2);
if tmp < 1e-4
    q_tilt = [0; 1; 0; 0];
    q_tors = [1; 0; 0; 0];
else
    q_tilt = [tmp; 
            (q(1) * q(2) - q(3) * q(4)) / tmp;
            (q(1) * q(3) + q(2) * q(4)) / tmp;
            0];
    q_tors = [q(1) / tmp; 0; 0; q(4) / tmp];
end

q_tilt = q_tilt / norm(q_tilt);
q_tors = q_tors / norm(q_tors);

q_tilt = q_tilt .* [1; -1; -1; -1]; 
q_tors = q_tors .* [1; -1; -1; -1]; 


cos_half_theta = q_tilt(1);
if abs(cos_half_theta - 1.0) < eps
    tilt = [0; 0];
else
    sin_half_theta = sqrt(q_tilt(2)^2 + q_tilt(3)^2);
    theta = 2.0 * atan2(sin_half_theta, cos_half_theta);
    tilt_axis = [q_tilt(2);q_tilt(3)];
    tilt_axis = tilt_axis / norm(tilt_axis);
    tilt = theta * tilt_axis;
end
tors = 2.0 * atan2(q_tors(4), q_tors(1));
